simulink model "PID_LoadCell_Magnet"  (Simulink 8.9)
settings: Solver=ode3  StartTime=0.0  StopTime=inf  FixedStep=0.001  RelTol=1e-3  EnableMultiTasking=on
libraries: slrtlib x4, xpcquanserlib x3, dsparch4 x2
settings Model: Creator=Ninad  LastModifiedBy=Rorro  SimulationMode=external
settings SolverCC: EnableConcurrentExecution=on
settings OptimizationCC: BlockReduction=off  OptimizeBlockIOStorage=off  BufferReuse=off  GlobalBufferReuse=off  ExpressionFolding=off  ExpressionDepthLimit=2147483647  LocalBlockOutputs=off
settings DebuggingCC: SolverPrmCheckMsg=warning
settings HardwareCC: ProdIntDivRoundTo=Zero  ProdEndianess=LittleEndian  ProdLongLongMode=on  ProdHWDeviceType=Generic->32-bit x86 compatible
settings RTWCC: SystemTargetFile=slrt.tlc  TemplateMakefile=slrt_default_tmf  Description=Simulink Real-Time  CodeExecutionProfiling=on  RTWCompilerOptimization=on
settings SimulinkRealTimeCC: GeneratePreprocessorConditionals=Disable all
settings ConfigComp: CovSFcnEnable=off

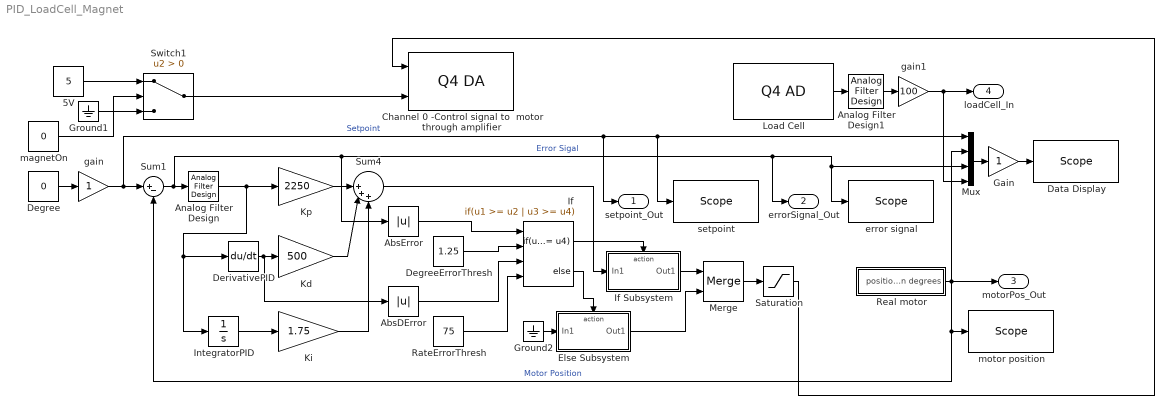
== system PID_LoadCell_Magnet ==
  5V : Constant  Value=5
  AbsDError : Abs
  AbsError : Abs
  Analog Filter Design : dsparch4/Analog Filter Design  method=Butterworth  filttype=Lowpass  N=1  Wlo=17  Whi=80  Rp=2  Rs=40
  Analog Filter Design1 : dsparch4/Analog Filter Design  method=Butterworth  filttype=Lowpass  N=1  Wlo=60  Whi=80  Rp=2  Rs=40
  "Channel 0 -Control signal to  motor through amplifier " : xpcquanserlib/D//A/Q4 DA   channel=[1:2]  range=[-10]  simul=off  reset=[1]  initValue=[0]  sampleTime=.001  slot=-1
      settings: SourceProductName=Simulink Real-Time  SourceProductBaseCode=XP
  Data Display : slrtlib/Displays and Logging/Scope   scopeno=3  scopetype=Target  autostart=on  viewmode=Numerical  formatstr="'Setpoint        %3.2f,Motor Position  %3.2f,Error Signal    %3.2f,Load Cell (V)    %4.3f'"  grid=on  ylimits=[0,170]  nosamples=200  noprepostsamples=0  interleave=10  triggermode=FreeRun  triggersignal=1  trigsignalfromport=off  triggerlevel=0.0  triggerslope=Either  triggerscope=1  triggersample=0  filename=data.dat  mode=Lazy  writesize=512  autorestart=off  dynamicfilemode=off  maxwritefilesize=512*1024^2
  Degree : Constant  Value=0
  DegreeErrorThresh : Constant  Value=1.25
  DerivativePID : Derivative
  Else Subsystem : Subsystem  TreatAsAtomicUnit=on
  Gain : Gain
  Ground1 : Ground
  Ground2 : Ground
  If : If  NumInputs=4  IfExpression=u1 >= u2 | u3 >= u4
  If Subsystem : Subsystem  TreatAsAtomicUnit=on
  IntegratorPID : Integrator
  Kd : Gain  Gain=500
  Ki : Gain  Gain=1.75
  Kp : Gain  Gain=2250
  Load Cell : xpcquanserlib/A//D/Q4 AD  channel=[1]  sampleTime=0.001  slot=-1
      settings: SourceProductName=Simulink Real-Time  SourceProductBaseCode=XP
  Merge : Merge
  Mux : Mux
  RateErrorThresh : Constant  Value=75
  Real motor : Subsystem
  Saturation : Saturate  UpperLimit=5  LowerLimit=-5
  Sum1 : Sum  Inputs=|+-
  Sum4 : Sum  Inputs=||+++
  Switch1 : Switch  Criteria=u2 > Threshold
  error signal : slrtlib/Displays and Logging/Scope   scopeno=2  scopetype=Target  autostart=on  viewmode=Graphical rolling  formatstr='%15.6f'  grid=on  ylimits=[-180,180]  nosamples=500  noprepostsamples=0  interleave=10  triggermode=FreeRun  triggersignal=1  trigsignalfromport=off  triggerlevel=0.0  triggerslope=Either  triggerscope=1  triggersample=0  filename=data.dat  mode=Lazy  writesize=512  autorestart=off  dynamicfilemode=off  maxwritefilesize=512*1024^2
  gain : Gain
  gain1 : Gain  Gain=100
  magnetOn : Constant  Value=0
  motor position : slrtlib/Displays and Logging/Scope   scopeno=7  scopetype=Target  autostart=on  viewmode=Graphical rolling  formatstr='%15.6f'  grid=on  ylimits=[-180,180]  nosamples=500  noprepostsamples=0  interleave=10  triggermode=FreeRun  triggersignal=1  trigsignalfromport=off  triggerlevel=0.0  triggerslope=Either  triggerscope=1  triggersample=0  filename=data.dat  mode=Lazy  writesize=512  autorestart=off  dynamicfilemode=off  maxwritefilesize=512*1024^2
  setpoint : slrtlib/Displays and Logging/Scope   scopeno=1  scopetype=Target  autostart=on  viewmode=Graphical rolling  formatstr='%15.6f'  grid=on  ylimits=[-180,180]  nosamples=500  noprepostsamples=0  interleave=10  triggermode=FreeRun  triggersignal=1  trigsignalfromport=off  triggerlevel=0.0  triggerslope=Either  triggerscope=1  triggersample=0  filename=data.dat  mode=Lazy  writesize=512  autorestart=off  dynamicfilemode=off  maxwritefilesize=512*1024^2
  setpoint_Out : Outport
  errorSignal_Out : Outport  Port=2
  motorPos_Out : Outport  Port=3
  loadCell_In : Outport  Port=4
  wires:
  Kd/1 -> Sum4/2
  DerivativePID/1 -> AbsDError/1, Kd/1
  IntegratorPID/1 -> Ki/1
  Ki/1 -> Sum4/3
  gain/1 -> Sum1/1, Mux/1, setpoint/1, setpoint_Out/1  "Setpoint"
  Degree/1 -> gain/1
  Real motor/1(position in degrees) -> Sum1/2, motor position/1, motorPos_Out/1, Mux/2  "Motor Position"
  Gain/1 -> Data Display/1
  Mux/1 -> Gain/1
  Sum1/1 -> AbsError/1, error signal/1, Mux/3, errorSignal_Out/1, Analog Filter Design/1  "Error Sigal"
  Else Subsystem/1(Out1) -> Merge/2
  If Subsystem/1(Out1) -> Merge/1
  Ground2/1 -> Else Subsystem/1(In1)
  AbsError/1 -> If/1
  AbsDError/1 -> If/3
  DegreeErrorThresh/1 -> If/2
  RateErrorThresh/1 -> If/4
  If/1 -> If Subsystem/Action
  If/2 -> Else Subsystem/Action
  Kp/1 -> Sum4/1
  Sum4/1 -> If Subsystem/1(In1)
  5V/1 -> Switch1/1
  magnetOn/1 -> Switch1/2
  Ground1/1 -> Switch1/3
  Switch1/1 -> "Channel 0 -Control signal to  motor through amplifier "/2
  Merge/1 -> Saturation/1
  Saturation/1 -> "Channel 0 -Control signal to  motor through amplifier "/1
  Load Cell/1 -> Analog Filter Design1/1
  Analog Filter Design/1 -> DerivativePID/1, IntegratorPID/1, Kp/1
  Analog Filter Design1/1 -> gain1/1
  gain1/1 -> Mux/4, loadCell_In/1

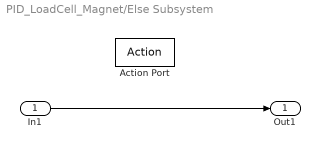
== system PID_LoadCell_Magnet/Else Subsystem ==
  In1 : Inport
  Action Port : ActionPort  ActionType=else
  Out1 : Outport
  wires:
  In1/1 -> Out1/1

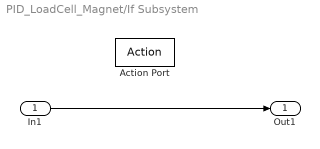
== system PID_LoadCell_Magnet/If Subsystem ==
  In1 : Inport
  Action Port : ActionPort  ActionType=then
  Out1 : Outport
  wires:
  In1/1 -> Out1/1

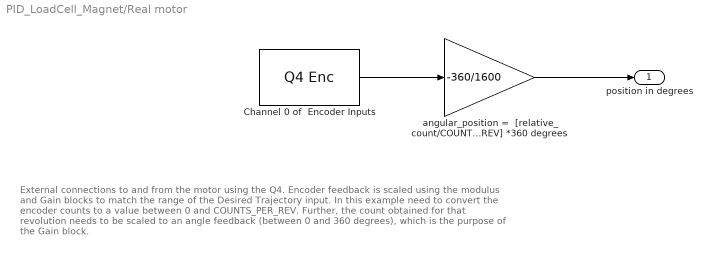
== system PID_LoadCell_Magnet/Real motor ==
  note: External connections to and from the motor using the Q4.
      |
      | Encoder feedback is scaled using the modulus and Gain blocks to
      | match the range of the Desired Trajectory input.
      |
      | In this example need to convert the encoder counts to a value between 0 and COUNTS_PER_REV.
      | Further, the count obtained for that revolution needs to be scaled to an angle feedback (between
      | 0 and 360 degrees), which is the purpose of the Gain block.
  "Channel 0 of  Encoder Inputs " : xpcquanserlib/Incremental Encoder/Q4 Enc   channel=[1]  initialCount=[0]  prescale=[1]  quadrature=[4]  mode=[0]  synchronousIndex=[0]  indexPolarity=[0]  preserveCounts=[0]  sampleTime=.001  slot=-1
      settings: SourceProductName=Simulink Real-Time  SourceProductBaseCode=XP
  angular_position =  [relative_count/COUNTS_PER_REV] *360 degrees : Gain  Gain=-360/1600
  position in degrees : Outport
  wires:
  angular_position =  [relative_count/COUNTS_PER_REV] *360 degrees/1 -> position in degrees/1
  "Channel 0 of  Encoder Inputs "/1 -> angular_position =  [relative_count/COUNTS_PER_REV] *360 degrees/1
